simulink model "HFI"  (R2023a)
settings: Solver=FixedStepDiscrete  StartTime=0.0  StopTime=10.0  RelTol=1e-3
model workspace (MATLAB code in the model file):
  | cmdLim = Simulink.Parameter;
  | cmdLim.Value = 15;
  | cmdLim.Description = 'Limit for controlling the maximum surface command angle.';
  | cmdLim.Min = 0;
  | cmdLim.Max = 90;
  | cmdLim.DocUnits = 'deg';
  | 
  | dispGain = Simulink.Parameter;
  | dispGain.Value = 0.75;
  | dispGain.Description = 'Gain applied to the displacement error.';
  | dispGain.Min = 0;
  | dispGain.Max = [];
  | dispGain.DocUnits = 'deg/sec/deg';
  | 
  | dispLim = Simulink.Parameter;
  | dispLim.Value = 30;
  | dispLim.Description = 'Limit for controlling the maximum commanded angle.';
  | dispLim.Min = 0;
  | dispLim.Max = 180;
  | dispLim.DocUnits = 'deg';
  | 
  | intGain = Simulink.Parameter;
  | intGain.Value = 0.5;
  | intGain.Description = 'Gain applied to the integral error.';
  | intGain.Min = 0;
  | intGain.Max = [];
  | intGain.DocUnits = 'deg/sec/deg/sec';
  | 
  | intLim = Simulink.Parameter;
  | intLim.Value = 5;
  | intLim.Description = 'Limit for controlling the maximum commanded angle.';
  | intLim.Min = 0;
  | intLim.Max = 90;
  | intLim.DocUnits = 'deg';
  | 
  | rateGain = Simulink.Parameter;
  | rateGain.Value = 2;
  | rateGain.Description = 'Gain applied to the rate error.';
  | rateGain.Min = 0;
  | rateGain.Max = [];
  | rateGain.DocUnits = 'deg/deg/sec';
  | 
  | rateLim = Simulink.Parameter;
  | rateLim.Value = 6;
  | rateLim.Description = 'Limit for controlling the maximum commanded angle.';
  | rateLim.Min = 0;
  | rateLim.Max = 180;
  | rateLim.DocUnits = 'deg/sec';
  | 
  | hdgGain = Simulink.Parameter;
  | hdgGain.Value = 0.015;
undefined symbols (not defined in the file): HFI_Status
libraries: simulink x1
settings Model: RequirementInfo={} %GIDa_fe9045fd_0412_4b6e_8206_617cc20e6fde  DataDictionary=HFI_Merge.sldd  Creator=洲  LastModifiedBy=洲
settings SolverCC: AlgebraicLoopSolver=TrustRegion  AutoInsertRateTranBlk=on
settings DataIOCC: SaveOutput=off  SignalLogging=off  DSMLogging=off  SaveTime=off
settings OptimizationCC: DefaultParameterBehavior=Inlined  UseDivisionForNetSlopeComputation=on  GainParamInheritBuiltInType=on  UseFloatMulNetSlope=on  UseSpecifiedMinMax=on  InlineInvariantSignals=on  EnhancedBackFolding=on  PassReuseOutputArgsAs=Individual arguments  ZeroExternalMemoryAtStartup=off  ZeroInternalMemoryAtStartup=off  NoFixptDivByZeroProtection=on  EfficientFloat2IntCast=on  LifeSpan=1  OptimizeBlockOrder=speed  DifferentSizesBufferReuse=on  OptimizationCustomize=off  EfficientTunableParamExpr=on
settings DebuggingCC: AllowSymbolicDim=off  SFUnexpectedBacktrackingDiag=warning  SFNoUnconditionalDefaultTransitionDiag=warning  SFExecutionAtInitializationDiag=none  ArithmeticOperatorsInVariantConditions=warning
settings HardwareCC: ProdLongLongMode=on
settings SFSimCC: MATLABDynamicMemAlloc=off
settings RTWCC: Description=Embedded Coder  SystemTargetFile=ert.tlc  TemplateMakefile=ert_default_tmf  BuildConfiguration=Faster Runs  DataTypeReplacement=CDataTypesFixedWidth
settings CodeAppCC: ForceParamTrailComments=on  IgnoreCustomStorageClasses=off  OperatorAnnotations=on  SimulinkDataObjDesc=on  SFDataObjDesc=on  CustomSymbolStrGlobalVar=rt$N$M  CustomSymbolStrType=$N$M  CustomSymbolStrFcn=$N$M$F  CustomSymbolStrMacro=$N$M  InsertBlockDesc=on  EnableCustomComments=on  ReqsInCode=on
settings ERTTargetCC: TargetLangStandard=C99 (ISO)  UtilityFuncGeneration=Shared location  MultiwordLength=2048  GenerateSampleERTMain=on  IncludeMdlTerminateFcn=off  CombineSignalStateStructs=on  SuppressErrorStatus=on  SupportAbsoluteTime=off  SupportNonFinite=off  SupportComplex=off  InlinedParameterPlacement=NonHierarchical  ERTCustomFileTemplate=example_file_process.tlc  ERTFilePackagingFormat=CompactWithDataFile
settings ConfigComp: CovScope=ReferencedModels  CovSaveName=covdata_rollAP  CovMetricSettings=dcmtrwe  CovHTMLOptions=-sRT=1 -aTS=1 -bRG=1 -bTC=1 -hTR=1 -nFC=0 -scm=1 -bcm=1 -xEv=0  CovSaveCumulativeToWorkspaceVar=on  CovSaveSingleToWorkspaceVar=on  CovCumulativeVarName=covCumulativeData_rollAP  CovReportOnPause=off  CovExternalEMLEnable=off  CovSFcnEnable=off

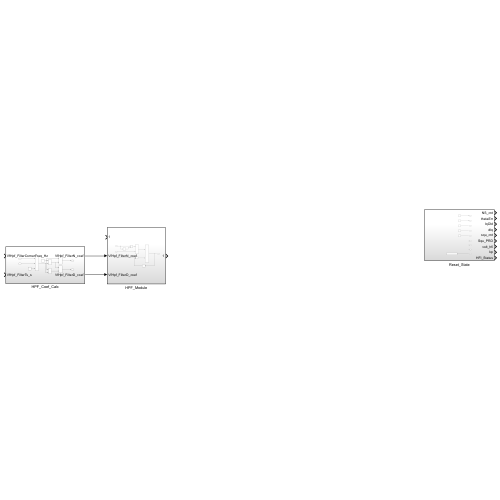
[thumbnail: Simulink's stored preview of the top-level diagram]
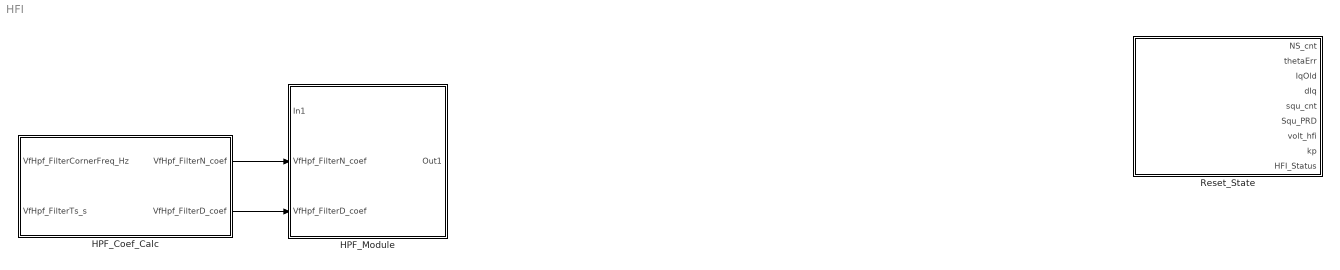
== system HFI ==
  HPF_Coef_Calc : Subsystem
  HPF_Module : Subsystem
  Reset_State : Subsystem
  wires:
  HPF_Coef_Calc/1(VfHpf_FilterN_coef) -> HPF_Module/2(VfHpf_FilterN_coef)
  HPF_Coef_Calc/2(VfHpf_FilterD_coef) -> HPF_Module/3(VfHpf_FilterD_coef)

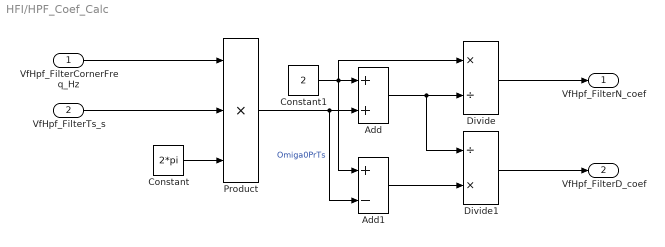
== system HFI/HPF_Coef_Calc ==
  VfHpf_FilterCornerFreq_Hz : Inport
  VfHpf_FilterTs_s : Inport  Port=2
  Add : Sum
  Add1 : Sum  Inputs=+-
  Constant : Constant  Value=2*pi  OutDataTypeStr=single
  Constant1 : Constant  Value=2  OutDataTypeStr=single
  Divide : Product  Inputs=*/
  Divide1 : Product  Inputs=/*
  Product : Product  Inputs=3
  VfHpf_FilterN_coef : Outport
  VfHpf_FilterD_coef : Outport  Port=2
  wires:
  VfHpf_FilterCornerFreq_Hz/1 -> Product/1
  VfHpf_FilterTs_s/1 -> Product/2
  Constant/1 -> Product/3
  Product/1 -> Add1/2, Add/2  "Omiga0PrTs"
  Constant1/1 -> Add1/1, Divide/1, Add/1
  Add/1 -> Divide1/1, Divide/2
  Divide/1 -> VfHpf_FilterN_coef/1
  Add1/1 -> Divide1/2
  Divide1/1 -> VfHpf_FilterD_coef/1

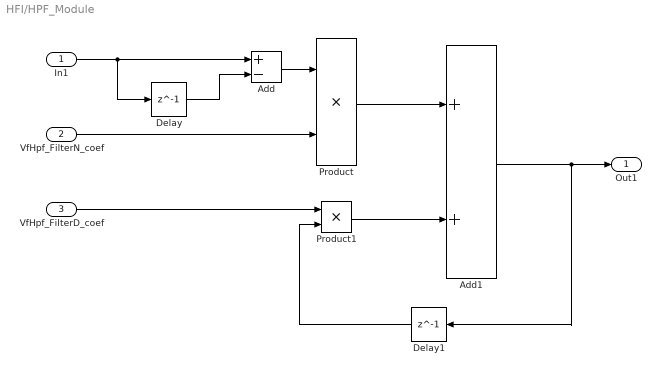
== system HFI/HPF_Module ==
  In1 : Inport
  VfHpf_FilterN_coef : Inport  Port=2
  VfHpf_FilterD_coef : Inport  Port=3
  Add : Sum  Inputs=+-
  Add1 : Sum
  Delay : Delay  DelayLength=1
  Delay1 : Delay  DelayLength=1
  Product : Product
  Product1 : Product
  Out1 : Outport
  wires:
  In1/1 -> Delay/1, Add/1
  Delay/1 -> Add/2
  Add/1 -> Product/1
  VfHpf_FilterN_coef/1 -> Product/2
  Product/1 -> Add1/1
  Add1/1 -> Delay1/1, Out1/1
  VfHpf_FilterD_coef/1 -> Product1/1
  Product1/1 -> Add1/2
  Delay1/1 -> Product1/2

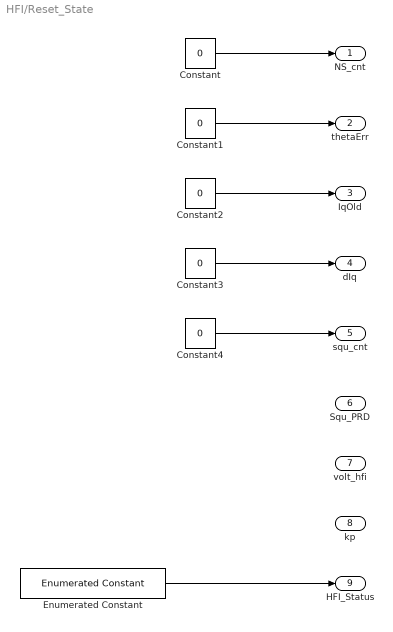
== system HFI/Reset_State ==
  Constant{,1..4} (5 alike) : Constant  Value=0  OutDataTypeStr=single
  Enumerated Constant : simulink/Sources/Enumerated Constant  OutDataTypeStr=Enum: HFI_Status  Value=HFI_Status.HFI_IPD_STATE  SampleTime=inf
  NS_cnt : Outport
  thetaErr : Outport  Port=2
  IqOld : Outport  Port=3
  dIq : Outport  Port=4
  squ_cnt : Outport  Port=5
  Squ_PRD : Outport  Port=6
  volt_hfi : Outport  Port=7
  kp : Outport  Port=8
  HFI_Status : Outport  Port=9
  wires:
  Constant/1 -> NS_cnt/1
  Constant2/1 -> IqOld/1
  Constant1/1 -> thetaErr/1
  Constant3/1 -> dIq/1
  Constant4/1 -> squ_cnt/1
  Enumerated Constant/1 -> HFI_Status/1
